simulink model "minsnap_traj_ex1"  (R2023b)
settings: Solver=VariableStepAuto  StartTime=0.0  StopTime=5  RelTol=1e-3
libraries: shareduavrstlib x1, simulink x1
settings Model: Creator=The MathWorks, Inc.  LastModifiedBy=Dz
settings SolverCC: MaxZcPerStep=1
settings ModelReferenceCC: EnableRefExpFcnMdlSchedulingChecks=on

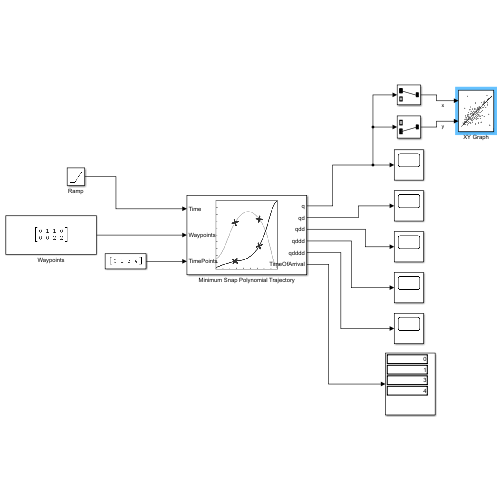
[thumbnail: Simulink's stored preview of the top-level diagram]
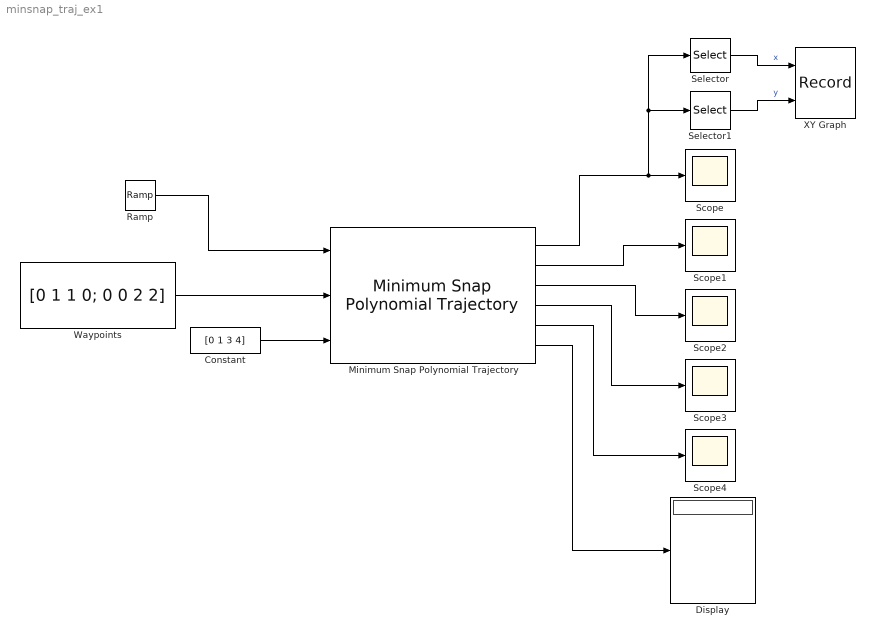
== system minsnap_traj_ex1 ==
  Constant : Constant  Value=[0 1 3 4]
  Display : Display
  Minimum Snap Polynomial Trajectory : shareduavrstlib/Minimum Snap Polynomial Trajectory  ShowBCInputPort=off  ShowPolynomialCoefs=off  ShowStatusOutputPort=off  TimeAllocation=off  TimeWeight=100  MinSegmentTime=0.1  MaxSegmentTime=1  MaxIteration=1500  MaxTime=10  SimulateUsing=Interpreted execution
  Ramp : simulink/Sources/Ramp  slope=1  start=0  InitialOutput=0
  Scope{,1..4} (5 alike) : Scope
  Selector : Selector  InputPortWidth=2  IndexOptions=Index vector (dialog)  Indices=1  OutputSizes=1
  Selector1 : Selector  InputPortWidth=2  IndexOptions=Index vector (dialog)  Indices=2  OutputSizes=1
  Waypoints : Constant  Value=[0 1 1 0; 0 0 2 2]
  XY Graph : Record  FileSettingsInternal="{\"entries\":[{\"content\":{\"excelSettings\":{\"content\":{},\"type\":\"Streamout.ExcelSettings\"}},\"type\":\"Streamout.FileSettingStorage\",\"uuid\":\"\"}],\"packageUris\":[\"http:\\/\\/schema.mathworks.com\\/mf0\\/streamout_blocks\\/R2020a\"],\"version\":\"1.0\"}"  Layout=[1 1]  SignalsInternal="{\"entries\":[{\"content\":{\"signals\":[{\"content\":{\"blockPath\":[],\"dimensions\":[1,1],\"domain\":\"\",\"lineColor\":\"#77ac30\",\"plots\":[1],\"port\":1,\"sid\":[\"\"],\"signalID\":498,\"signalName\":\"x\"},\"type\":\"RecordBlkView.Signal\",\"uuid\":\"\"},{\"content\":{\"blockPath\":[],\"dimensions\":[1,1],\"domain\":\"\",\"lineColor\":\"#4dbeee\",\"plots\":[1],\"port\":2,\"sid\":[\"\"],\"signalID\":502,\"signalName\":\"y\"},\"type\":\"RecordBlkView.Signal\",\"uuid\":\"\"}]},\"type\":\"RecordBlkView.InputSignals\",\"uuid\":\"\"}],\"packageUris\":[\"http:\\/\\/schema.mathworks.com\\/mf0\\/streamout_blocks\\/R2020a\"],\"version\":\"1.0\"}"  VisualizationBindings="{\"xyplotplugin\":{\"info\":[{\"series\":[{\"bindingParametersList\":[{\"parameter\":\"X-Axis\",\"signalID\":498,\"signalName\":\"x\"},{\"parameter\":\"Y-Axis\",\"signalID\":502,\"signalName\":\"y\"}],\"seriesID\":9148}],\"subplotID\":1}]}}"  CompatibilityTag=XY  st=-1
  wires:
  Minimum Snap Polynomial Trajectory/3 -> Scope2/1
  Waypoints/1 -> Minimum Snap Polynomial Trajectory/2
  Minimum Snap Polynomial Trajectory/1 -> Selector1/1, Selector/1, Scope/1
  Selector/1 -> XY Graph/1  "x"
  Selector1/1 -> XY Graph/2  "y"
  Minimum Snap Polynomial Trajectory/2 -> Scope1/1
  Ramp/1 -> Minimum Snap Polynomial Trajectory/1
  Constant/1 -> Minimum Snap Polynomial Trajectory/3
  Minimum Snap Polynomial Trajectory/4 -> Scope3/1
  Minimum Snap Polynomial Trajectory/6 -> Display/1
  Minimum Snap Polynomial Trajectory/5 -> Scope4/1
